simulink model "forward_2017a"  (R2017a)
settings: Solver=VariableStepAuto  StartTime=0.0  StopTime=10.0  RelTol=1e-3
values from neighbouring files (symbols this model uses):
  k1_m = 600    [Calculations.m]
  k2_m = 500    [Calculations.m]
  K_thruster = P1 / U1    (= 24.525)    [Calculations.m]
  lambda11 = 12.72    [Calculations.m]
  m = 300    [Calculations.m]
  T_thruster = 0.3    [Calculations.m]
undefined symbols (not defined in the file or in its folder): Cx1, Cx2
settings Model: Creator=corsair  LastModifiedBy=corsair
settings DataIOCC: ReturnWorkspaceOutputs=on
settings SFSimCC: SimUseLocalCustomCode=on
settings RTWCC: RTWUseLocalCustomCode=on

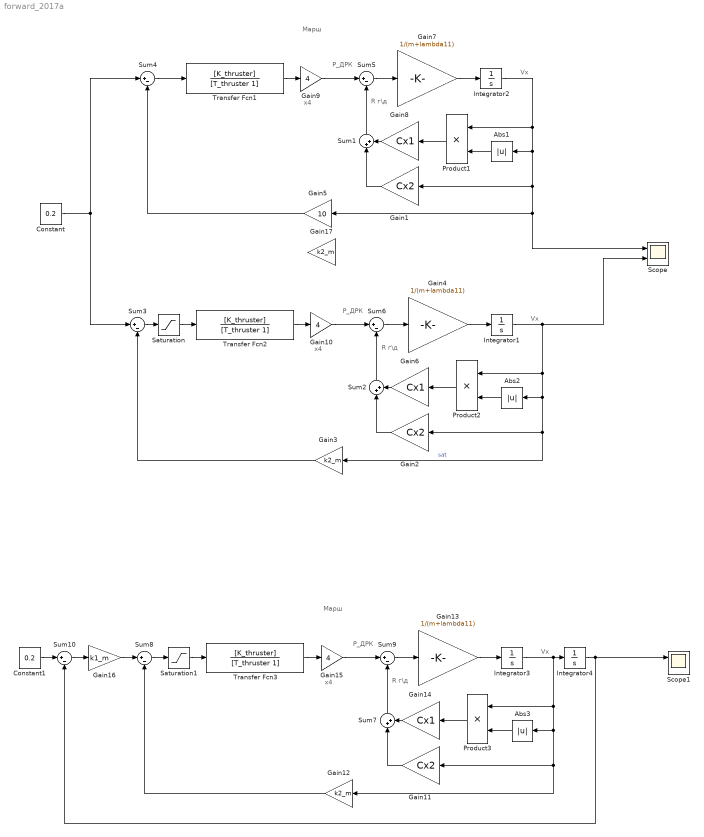
== system forward_2017a ==
  note: x4
  note: R г\д
  note: P_ДРК
  note: Марш
  note: Vx
  note: x4
  note: R г\д
  note: P_ДРК
  note: Vx
  note: x4
  note: R г\д
  note: P_ДРК
  note: Марш
  note: Vx
  Abs1 : Abs
  Abs2 : Abs
  Abs3 : Abs
  Constant : Constant  Value=0.2
  Constant1 : Constant  Value=0.2
  Gain1 : Gain  Gain=Cx2
  Gain10 : Gain  Gain=4
  Gain11 : Gain  Gain=Cx2
  Gain12 : Gain  Gain=k2_m
  Gain13 : Gain  Gain=1/(m+lambda11)
  Gain14 : Gain  Gain=Cx1
  Gain15 : Gain  Gain=4
  Gain16 : Gain  Gain=k1_m
  Gain17 : Gain  Gain=k2_m
  Gain2 : Gain  Gain=Cx2
  Gain3 : Gain  Gain=k2_m
  Gain4 : Gain  Gain=1/(m+lambda11)
  Gain5 : Gain  Gain=10
  Gain6 : Gain  Gain=Cx1
  Gain7 : Gain  Gain=1/(m+lambda11)
  Gain8 : Gain  Gain=Cx1
  Gain9 : Gain  Gain=4
  Integrator{1..4} (4 alike) : Integrator
  Product1 : Product
  Product2 : Product
  Product3 : Product
  Saturation : Saturate
  Saturation1 : Saturate
  Scope : Scope  NumInputPorts=2
  Scope1 : Scope  NumInputPorts=2
  Sum1 : Sum  Inputs=|++
  Sum{3..6,8..10} (7 alike) : Sum  Inputs=|+-
  Sum2 : Sum  Inputs=|++
  Sum7 : Sum  Inputs=|++
  Transfer Fcn1 : TransferFcn  Numerator=[K_thruster]  Denominator=[T_thruster 1]
  Transfer Fcn2 : TransferFcn  Numerator=[K_thruster]  Denominator=[T_thruster 1]
  Transfer Fcn3 : TransferFcn  Numerator=[K_thruster]  Denominator=[T_thruster 1]
  wires:
  Abs1/1 -> Product1/2
  Gain9/1 -> Sum5/1
  Integrator2/1 -> Scope/1, Gain5/1, Gain1/1, Abs1/1, Product1/1
  Gain7/1 -> Integrator2/1
  Sum5/1 -> Gain7/1
  Sum4/1 -> Transfer Fcn1/1
  Transfer Fcn1/1 -> Gain9/1
  Gain5/1 -> Sum4/2
  Product1/1 -> Gain8/1
  Gain8/1 -> Sum1/2
  Sum1/1 -> Sum5/2
  Gain1/1 -> Sum1/1
  Gain2/1 -> Sum2/1
  Sum2/1 -> Sum6/2
  Gain6/1 -> Sum2/2
  Product2/1 -> Gain6/1
  Gain3/1 -> Sum3/2
  Transfer Fcn2/1 -> Gain10/1
  Sum3/1 -> Saturation/1
  Sum6/1 -> Gain4/1
  Gain4/1 -> Integrator1/1
  Constant/1 -> Sum4/1, Sum3/1
  Integrator1/1 -> Product2/1, Abs2/1, Gain3/1, Gain2/1, Scope/2  "sat"
  Gain10/1 -> Sum6/1
  Abs2/1 -> Product2/2
  Saturation/1 -> Transfer Fcn2/1
  Gain11/1 -> Sum7/1
  Sum7/1 -> Sum9/2
  Gain14/1 -> Sum7/2
  Product3/1 -> Gain14/1
  Gain12/1 -> Sum8/2
  Transfer Fcn3/1 -> Gain15/1
  Sum9/1 -> Gain13/1
  Gain13/1 -> Integrator3/1
  Integrator3/1 -> Product3/1, Abs3/1, Gain11/1, Gain12/1, Integrator4/1
  Gain15/1 -> Sum9/1
  Abs3/1 -> Product3/2
  Constant1/1 -> Sum10/1
  Sum10/1 -> Gain16/1
  Gain16/1 -> Sum8/1
  Integrator4/1 -> Scope1/1, Sum10/2
  Saturation1/1 -> Transfer Fcn3/1
  Sum8/1 -> Saturation1/1
